simulink model "motorSimulation"  (R2020a)
settings: Solver=FixedStepAuto  StartTime=0.0  StopTime=15  FixedStep=0.002  RelTol=1e-3  EnableMultiTasking=on
libraries: simulink x2
settings Model: ExtModeTrigDuration=10000  Creator=KIMAIDE  LastModifiedBy=KIMAIDE
settings SolverCC: PositivePriorityOrder=on
settings DataIOCC: ReturnWorkspaceOutputs=off
settings OptimizationCC: LifeSpan=inf
settings DebuggingCC: ArithmeticOperatorsInVariantConditions=warning
settings SFSimCC: SimUseLocalCustomCode=off  CustomCodeUndefinedFunction=UseInterfaceOnly
settings RTWCC: Description=QUARC Win64 Target  SystemTargetFile=quarc_win64.tlc  TemplateMakefile=quarc_default_tmf  RTWUseLocalCustomCode=off
settings CodeAppCC: StateflowObjectComments=on
settings STFCustomTargetCC: TargetPreCompLibLocation=C:\PROGRA~3\QUARC\lib\2016a\win64\release  TargetLangStandard=C99 (ISO)  ConcurrentExecutionCompliant=on  GRTInterface=on  SystemTargetFile=quarc_win64.tlc
settings GRTTargetCC: TargetPreCompLibLocation=C:\PROGRA~3\QUARC\lib\2016a\win64\release  ParMdlRefBuildCompliant=off  CompOptLevelCompliant=off  CombineOutputUpdateFcns=off  MatFileLogging=off  CPPClassGenCompliant=off  GRTInterface=on  UseToolchainInfoCompliant=off  ExtMode=on  ExtModeMexFile=quarc_comm
settings ConfigComp: CovMetricSettings=dswe

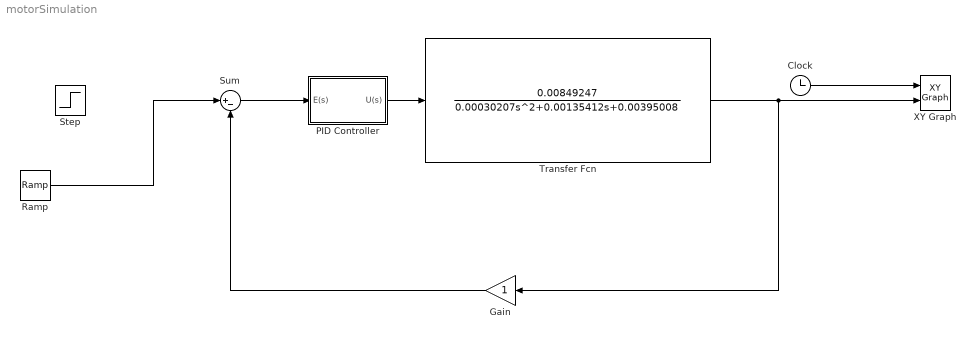
== system motorSimulation ==
  Clock : Clock
  Gain : Gain
  PID Controller : Subsystem
  Ramp : simulink/Sources/Ramp  slope=-1  start=0  InitialOutput=5
  Step : Step  Time=0  SampleTime=0
  Sum : Sum  Inputs=|+-
  Transfer Fcn : TransferFcn  Numerator=[0.00849247]  Denominator=[0.00030207 0.00135412 0.00395008]
  XY Graph : simulink/Sinks/XY Graph  xmin=0  xmax=15  ymin=-10  ymax=10  st=-1
  wires:
  Transfer Fcn/1 -> XY Graph/2, Gain/1
  PID Controller/1(U(s)) -> Transfer Fcn/1
  Sum/1 -> PID Controller/1(E(s))
  Gain/1 -> Sum/2
  Clock/1 -> XY Graph/1
  Ramp/1 -> Sum/1

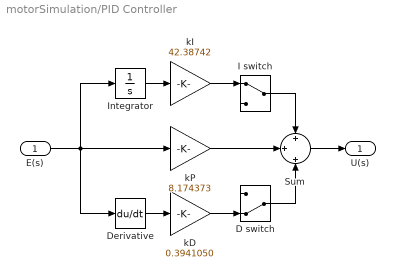
== system motorSimulation/PID Controller ==
  E(s) : Inport
  D switch : ManualSwitch  CurrentSetting=0
  Derivative : Derivative
  I switch : ManualSwitch
  Integrator : Integrator
  Sum : Sum  Inputs=+|+|+
  kD : Gain  Gain=0.3941050  ParamMin=[0]  ParamMax=[5]
  kI : Gain  Gain=42.38742  ParamMin=[0]  ParamMax=[100]
  kP : Gain  Gain=8.174373  ParamMin=[0]  ParamMax=[200]
  U(s) : Outport  VectorParamsAs1DForOutWhenUnconnected=off
  wires:
  E(s)/1 -> kP/1, Integrator/1, Derivative/1
  kP/1 -> Sum/2
  Sum/1 -> U(s)/1
  Derivative/1 -> kD/1
  Integrator/1 -> kI/1
  kI/1 -> I switch/1
  I switch/1 -> Sum/1
  kD/1 -> D switch/2
  D switch/1 -> Sum/3
